simulink model "c221007_FCEV_CDCS"  (R2022b)
settings: Solver=ode4  StartTime=1  StopTime=size(Driving_cycle_v_kmph,1)  FixedStep=Auto  RelTol=1e-3  EnableMultiTasking=on
values from neighbouring files (symbols this model uses):
  Bat_eff_chg_average = 0.969    [FCEV_original_data.mat]
  Bat_eff_dis_average = 0.9632    [FCEV_original_data.mat]
  Bat_end_of_life_percent = 20    [FCEV_original_data.mat]
  Bat_I_chg_max = -120    [FCEV_original_data.mat]
  Bat_I_dis_max = 200    [FCEV_original_data.mat]
  Bat_nom_Ic = 2.5    [FCEV_original_data.mat]
  Bat_nom_SOC = 0.35    [FCEV_original_data.mat]
  Bat_nom_temp_oC = 25    [FCEV_original_data.mat]
  Bat_num_pa = 9    [FCEV_original_data.mat]
  Bat_num_se = 97    [FCEV_original_data.mat]
  Bat_ori_C1_chg_F = [397.526659684 455.660832136 435.08783522 460.845064365 457.605812374 417.289828504 416.373906992 359.741413056 321.561704819 1109.14132554 1165.67733205 1135.97600211 ... (72 elements, 9x8)]    [FCEV_original_data.mat]
  Bat_ori_C1_dis_F = [187.121968588 287.083505726 346.448009002 395.529439835 387.517274826 389.973134196 432.856765051 486.92921923 512.158935268 425.990733989 614.68708868 771.472592368 ... (72 elements, 9x8)]    [FCEV_original_data.mat]
  Bat_ori_C2_chg_F = [8748.48589695 7773.35875681 9404.86567646 8934.73981058 8290.58671366 7592.78422269 7759.44623103 7396.59043829 6151.35152293 16187.7227039 11721.8480541 13157.8579836 ... (72 elements, 9x8)]    [FCEV_original_data.mat]
  Bat_ori_C2_dis_F = [2939.81325553 4590.73311898 5504.93546413 5887.5077374 6534.37836712 7765.46899768 10584.7751706 10372.0508438 9238.72693885 5207.86390693 7911.43744944 8879.62137571 ... (72 elements, 9x8)]    [FCEV_original_data.mat]
  Bat_ori_cap_max_Ah = 20.7    [Config_c221218.m]    (also in Config_c230117.m; Config_c230321.m; FCEV_original_data.mat)
  Bat_ori_dUdt4 = [-0.303773584906 -0.249056603774 -0.115094339623 -0.0396226415094 0.0396226415094 0.0641509433962 0.107547169811 0.111320754717 0.0415094339623 0.0547169811321 0.130188679245]    [FCEV_original_data.mat]
  Bat_ori_R0_chg_O = [0.0771669453735 0.0731809311402 0.0726556782939 0.0729965156794 0.0731758310684 0.0742031005051 0.0721266921026 0.0714211058078 0.0714186176143 0.0374124505155 0.0354566732504 0.0345430657188 ... (72 elements, 9x8)]    [FCEV_original_data.mat]
  Bat_ori_R0_dis_O = [0.0819458671157 0.0812429476608 0.0803749674507 0.0805513601722 0.0838629023857 0.0850797840015 0.0829875518672 0.0826388888889 0.0812514106148 0.0428124986417 0.0424658903711 0.0428572670451 ... (72 elements, 9x8)]    [FCEV_original_data.mat]
  Bat_ori_R1_chg_O = [0.114339870884 0.105392753268 0.104421193553 0.109821896183 0.114868279838 0.123333154908 0.129174812826 0.149917249373 0.174896487845 0.0420560161846 0.0390948352938 0.0370122837364 ... (72 elements, 9x8)]    [FCEV_original_data.mat]
  Bat_ori_R1_dis_O = [0.304806399643 0.213604089624 0.171463520004 0.151183840498 0.140630862434 0.128795299077 0.116857791733 0.112567113582 0.106368362501 0.0943235089866 0.0730697254134 0.0611414736086 ... (72 elements, 9x8)]    [FCEV_original_data.mat]
  Bat_ori_R2_chg_O = [0.134518959939 0.17565045702 0.161100627268 0.189032232545 0.205639040497 0.226170473035 0.223651875822 0.181765694192 0.212966950836 0.073628872144 0.0788540822416 0.0792414571734 ... (72 elements, 9x8)]    [FCEV_original_data.mat]
  Bat_ori_R2_dis_O = [0.354968099904 0.285293035102 0.286338708953 0.298763853987 0.248762838155 0.178586175471 0.129047399775 0.188406991173 0.174494800676 0.131839238891 0.123225430215 0.132069033134 ... (72 elements, 9x8)]    [FCEV_original_data.mat]
  Bat_ori_SOC2 = [0 0.001 0.002 0.003 0.004 0.005 0.006 0.007 0.008 0.009 0.01 0.011 ... (1001 elements, 1x1001)]    [FCEV_original_data.mat]
  Bat_ori_SOC4 = [-0.00598301069999 0.0920117618231 0.190864167279 0.289083557951 0.387343788287 0.485011843502 0.5850485992 0.678163031937 0.774810095565 0.876684636119 0.972739524626]    [FCEV_original_data.mat]
  Bat_ori_Uoc_chg_V = [2.4478 2.54923264342 2.6007 2.6383 2.66953057366 2.69636321708 2.7197 2.74042850391 2.75906114733 2.77619379074 2.792 2.80675907757 ... (1001 elements, 1x1001)]    [FCEV_original_data.mat]
  Bat_ori_Uoc_dis_V = [1.9998 2.03916768329 2.24724374236 2.39700902919 2.48767431602 2.5476 2.5882 2.6202 2.64771773167 2.6719 2.6933 2.71251566192 ... (1001 elements, 1x1001)]    [FCEV_original_data.mat]
  Bat_ori_Uoc_V = [2.2238 2.29420016335 2.42397187118 2.5176545146 2.57860244484 2.62198160854 2.65395 2.68031425195 2.7033894395 2.72404689537 2.74265 2.75963736975 ... (1001 elements, 1x1001)]    [FCEV_original_data.mat]
  Bat_single_capacity_nom_Ah = 2.3    [FCEV_original_data.mat]
  Bat_SOC_cs_max = 0.4    [FCEV_original_data.mat]
  Bat_SOC_cs_min = 0.2    [FCEV_original_data.mat]
  Bat_SOC_ini = 0.3    [Config_c22100601.m]    (also in Config_c22100701.m; FCEV_original_data.mat = 0.45)
  Bat_SOC_max = 0.9    [FCEV_original_data.mat]
  Bat_SOC_min = 0.3    [FCEV_original_data.mat]
  Bat_temp_amb_oC = 25    [FCEV_original_data.mat]
  Bat_temp_cool_oC = 25    [FCEV_original_data.mat]
  Bat_U_avg_V = Bat_num_se*mean(Bat_ori_Uoc_V)    [Config_c22100601.m]    (also in Config_c22100701.m)
  DCAC_eff = 0.95    [FCEV_original_data.mat]
  DCDC_ori_eff = [0.95 0.96 0.97 0.976 0.98 0.978 0.973 0.962]    [FCEV_original_data.mat]
  DCDC_ori_power_kW = [0 10 20 30 40 50 60 70]    [FCEV_original_data.mat]
  FC_fuel_mass_ini_kg = 10    [FCEV_original_data.mat]
  FC_ori_eff = [0.1 0.33 0.492 0.533 0.559 0.596 0.591 0.562 0.508]    [FCEV_original_data.mat]
  FC_ori_fuel_rate_gps = [0 0.0505050505051 0.0846883468835 0.117260787992 0.149075730471 0.279642058166 0.423011844332 0.593119810202 0.820209973753]    [FCEV_original_data.mat]
  FC_ori_power_kW = [0 2 5 7.5 10 20 30 40 50]    [FCEV_original_data.mat]
  FC_power_max_kW = 50    [FCEV_original_data.mat]
  FC_power_min_kW = 0    [FCEV_original_data.mat]
  MC_eff_brk_average = 0.810578512397    [FCEV_original_data.mat]
  MC_eff_dri_average = 0.810578512397    [FCEV_original_data.mat]
  MC_inertia = 0.06    [FCEV_original_data.mat]
  MC_ori_eff = [0.7 0.78 0.85 0.86 0.81 0.82 0.79 0.78 0.78 0.78 0.78 0.7 ... (231 elements, 11x21)]    [FCEV_original_data.mat]
  MC_ori_power_brk_req_kW = [0 -28.3912930389 -56.7825860779 -85.1738791168 -113.565172156 -141.956465195 -170.347758234 -198.739051273 -227.130344311 -255.52163735 -283.912930389 0 ... (121 elements, 11x11)]    [FCEV_original_data.mat]
  MC_ori_power_dri_req_kW = [0 0 0 0 0 0 0 0 0 0 0 0 ... (121 elements, 11x11)]    [FCEV_original_data.mat]
  MC_ori_spd_rpm = [0 1000 2000 3000 4000 5000 6000 7000 8000 9000 10000]    [FCEV_original_data.mat]
  MC_ori_trq_brk_max_Nm = [-271.1368 -271.1368 -271.1368 -237.5159 -178.1369 -142.4824 -118.7579 -101.8119 -89.0685 -79.172 -71.1734]    [FCEV_original_data.mat]
  MC_ori_trq_brk_Nm = [-271.136848522 -244.02316367 -216.909478817 -189.795793965 -162.682109113 -135.568424261 -108.454739409 -81.3410545565 -54.2273697044 -27.1136848522 0]    [FCEV_original_data.mat]
  MC_ori_trq_dri_max_Nm = [271.1368 271.1368 271.1368 237.5159 178.1369 142.4824 118.7579 101.8119 89.0685 79.172 71.1734]    [FCEV_original_data.mat]
  MC_ori_trq_dri_Nm = [0 27.1136848522 54.2273697044 81.3410545565 108.454739409 135.568424261 162.682109113 189.795793965 216.909478817 244.02316367 271.136848522]    [FCEV_original_data.mat]
  MC_ori_trq_Nm = [-271.136848522 -244.02316367 -216.909478817 -189.795793965 -162.682109113 -135.568424261 -108.454739409 -81.3410545565 -54.2273697044 -27.1136848522 0 27.1136848522 ... (21 elements, 1x21)]    [FCEV_original_data.mat]
  MC_power_max_kW = 75    [FCEV_original_data.mat]
  MC_spd_max_rpm = 10000    [FCEV_original_data.mat]
  MC_spd_min_rpm = 0    [FCEV_original_data.mat]
  MC_spd_scale = 1    [FCEV_original_data.mat]
  MC_trq_scale = 1    [FCEV_original_data.mat]
  MC_U_min_V = 120    [FCEV_original_data.mat]
  Road_u = 0.75    [FCEV_original_data.mat]
  S_r = floor(max(Sr_SOC_process(:,1))):-1:0    [Config_c22100601.m]    (also in Config_c22100701.m)
  Time_sample = 60    [Driving_cycle_recognition_data.mat]
  Trip_distance_total_km = sum(Driving_cycle_v_kmph(:,2)/3.6)/1000    [Config_c22100601.m]    (also in Config_c22100701.m)
  usd2rmb = 7.116    [Config_c22100601.m]    (also in Config_c22100701.m; Config_c221106.m = 6; Config_c221112.m = 6; Config_c221127.m = 6)
  Veh_air_density_kgpm2 = 1.2    [FCEV_original_data.mat]
  Veh_brk_front = [1 0.6 0.608 0.61 0.618 0.624 0.636 0.645 0.655]    [FCEV_original_data.mat]
  Veh_brk_z = [0.1 0.2 0.3 0.4 0.5 0.6 0.7 0.8 0.9]    [FCEV_original_data.mat]
  Veh_brk_z_max = 0.7    [FCEV_original_data.mat]
  Veh_brk_z_min = 0.1    [FCEV_original_data.mat]
  Veh_coeff_drag = 0.312    [FCEV_original_data.mat]
  Veh_coeff_roll = 0.00863    [FCEV_original_data.mat]
  Veh_final_drive_inertia = 0.1105    [FCEV_original_data.mat]
  Veh_final_drive_ratio = 3.47    [FCEV_original_data.mat]
  Veh_frontal_area_m2 = 2.06    [FCEV_original_data.mat]
  Veh_gravity_acc_ms2 = 9.81    [FCEV_original_data.mat]
  Veh_mass_cargo_kg = 113    [FCEV_original_data.mat]
  Veh_mass_curb_kg = 1157    [FCEV_original_data.mat]
  Veh_mech_eff = 0.9    [FCEV_original_data.mat]
  Veh_rotary_mass_conversion_factor = 1.05    [FCEV_original_data.mat]
  Veh_size_cg_height_m = 0.53    [FCEV_original_data.mat]
  Veh_wheel_inertia = 3.1039    [FCEV_original_data.mat]
  Veh_wheel_radius_m = 0.313    [FCEV_original_data.mat]
  Veh_wt_frac_front = 0.5    [FCEV_original_data.mat]
undefined symbols (not defined in the file or in its folder): alpha, Bat_ori_temp, Sr_e
libraries: neural x10
(part 5 of 5)

== system c221007_FCEV_CDCS/电池模型/Subsystem/Electrical Model1/Parameter Lookup2/Lookup Rs ==
  SOC : Inport
  T : Inport  Port=2
  Lookup Table (2-D) R0_c : Lookup2D  RowIndex=Bat_ori_SOC_chg  ColumnIndex=Bat_ori_temp_oC  Table=Bat_ori_R0_chg_O  SaturateOnIntegerOverflow=off  InputSameDT=off
  Lookup Table (2-D) R0_d : Lookup2D  RowIndex=Bat_ori_SOC_dis  ColumnIndex=Bat_ori_temp_oC  Table=Bat_ori_R0_dis_O  SaturateOnIntegerOverflow=off  InputSameDT=off
  Mux : Mux  Inputs=2
  R0 : Outport
  tag scope: Bat_R0_chg_O=global, Bat_R0_dis_O=global
  wires:
  Lookup Table (2-D) R0_d/1 -> Mux/1, [Bat_R0_dis_O]
  Lookup Table (2-D) R0_c/1 -> Mux/2, [Bat_R0_chg_O]
  SOC/1 -> Lookup Table (2-D) R0_c/1, Lookup Table (2-D) R0_d/1
  T/1 -> Lookup Table (2-D) R0_c/2, Lookup Table (2-D) R0_d/2
  Mux/1 -> R0/1

== system c221007_FCEV_CDCS/电池模型/Subsystem/Electrical Model1/Parameter Lookup2/Lookup Uoc ==
  SOC : Inport
  P : Inport  Port=2
  Switch : Switch  SaturateOnIntegerOverflow=off  InputSameDT=off
  VOC-chg : Lookup_n-D  NumberOfTableDimensions=1  BreakpointsForDimension1=Bat_ori_SOC2  BreakpointsForDimension2=Bat_ori_temp  Table=Bat_ori_Uoc_chg_V  InternalRulePriority=Speed  RndMeth=Simplest
  VOC-dischg : Lookup_n-D  NumberOfTableDimensions=1  BreakpointsForDimension1=Bat_ori_SOC2  BreakpointsForDimension2=Bat_ori_temp  Table=Bat_ori_Uoc_dis_V  InternalRulePriority=Speed  RndMeth=Simplest
  Uoc : Outport
  wires:
  SOC/1 -> VOC-chg/1, VOC-dischg/1
  VOC-chg/1 -> Switch/3
  VOC-dischg/1 -> Switch/1
  Switch/1 -> Uoc/1
  P/1 -> Switch/2

== system c221007_FCEV_CDCS/电池模型/Subsystem/Electrical Model1/SOC Calculation/CD//CS mode judgement ==
  note: 当前SOC
  SOC : Inport
  Constant2 : Constant  Value=Bat_SOC_min
  Logical Operator1 : Logic  Operator=NOT  AllPortsSameDT=off  OutDataTypeStr=boolean
  Relational Operator : RelationalOperator  OutDataTypeStr=boolean  InputSameDT=off
  Scope1 : Scope
  To Workspace2 : ToWorkspace  VariableName=Bat_charge_sustaining_on  SampleTime=-1
  tag scope: Bat_charge_sustaining_on=global
  wires:
  SOC/1 -> Relational Operator/1
  Constant2/1 -> Relational Operator/2
  Logical Operator1/1 -> Scope1/1, To Workspace2/1, [Bat_charge_sustaining_on]
  Relational Operator/1 -> Logical Operator1/1

== matlab function c221007_FCEV_CDCS/燃料电池模型/FcDegCountingSubSys/MATLAB Function4 ==
  data: u input; y output; usd2rmb input
function y = FcDegHl(u,usd2rmb)
alpha_h = 10;   %10e-6V/h
u_eol = 100000;   %10e-6V
p_stack = 50*93*usd2rmb;

y = (alpha_h*p_stack/u_eol)*u/3600;

== matlab function c221007_FCEV_CDCS/燃料电池模型/FcDegCountingSubSys/MATLAB Function5 ==
  data: u input; y output; usd2rmb input
function y = FcDegLl(u,usd2rmb)
alpha_l = 8.66;   %10e-6V/h
u_eol = 100000;   %10e-6V
p_stack = 50*93*usd2rmb;

y = (alpha_l*p_stack/u_eol)*u/3600;

== stateflow chart c221007_FCEV_CDCS/模式切换/Chart ==
  settings: sampleTime=1
  state Stop
    entry:Mode=0
  state Mode_B
    entry:Mode=1
  state Mode_FC
    entry:Mode=3
  state Mode_C21
    entry:Mode=2
  state Mode_C22
    entry:Mode=2
  state Mode_H
    entry:Mode=4
  state Mode_RB
    entry:Mode=5
  (default) -> Stop
  Mode_RB -> Stop [order 2] : [Bat_SOC > Bat_SOC_max]
  Stop -> (junction 123) : [PS_power_req_kW<0|PS_power_req_kW>0]
  (junction 123) -> Stop [order 5] : [PS_power_req_kW==0]
  (junction 123) -> Mode_B [order 4] : [PS_power_req_kW>0&PS_power_req_kW<=FC_power_min_kW]
  Mode_FC -> (junction 123) : [PS_power_req_kW<=FC_power_min_kW|PS_power_req_kW>FC_power_max_kW]
  (junction 123) -> Mode_FC [order 1] : [PS_power_req_kW>FC_power_min_kW&PS_power_req_kW<=FC_power_max_kW&Bat_SOC > Bat_SOC_max]
  Mode_B -> (junction 123) : [PS_power_req_kW<=0|PS_power_req_kW>FC_power_min_kW]
  (junction 123) -> Mode_C21 [order 6] : [PS_power_req_kW>0&PS_power_req_kW<=FC_power_min_kW&Bat_SOC<=Bat_SOC_min]
  Mode_C22 -> (junction 123) : [PS_power_req_kW<=FC_power_min_kW|PS_power_req_kW>FC_power_max_kW]
  (junction 123) -> Mode_C22 [order 7] : [PS_power_req_kW>FC_power_min_kW&PS_power_req_kW<=FC_power_max_kW&Bat_SOC <=Bat_SOC_max]
  Mode_C21 -> (junction 123) : [PS_power_req_kW<=0|PS_power_req_kW>FC_power_min_kW]
  Mode_RB -> (junction 123) [order 1] : [PS_power_req_kW>=0]
  (junction 123) -> Mode_RB [order 2] : [PS_power_req_kW<0]
  Mode_H -> (junction 123) : [PS_power_req_kW<=FC_power_max_kW]
  (junction 123) -> Mode_H [order 3] : [PS_power_req_kW>FC_power_max_kW]
  data: PS_power_req_kW input; Bat_SOC_min input; Bat_SOC_max input; FC_power_min_kW input; FC_power_max_kW input; Bat_SOC input; Mode output double
